simulink model "new16QAM"  (R2017b)
settings: Solver=VariableStepAuto  StartTime=0.0  StopTime=10.0  RelTol=1e-3
values from neighbouring files (symbols this model uses):
  Gain_lin = 10^(GdB/20)    [Microwave_Link.m]
  Var = 10^((N_dBm - 30)/10)    [Microwave_Link.m]
libraries: commblkcod2 x2, commdigbbndam3 x2, commchan3 x1, commsync2 x1, commsink2 x1, commrflib2 x1, commrandsrc3 x1
settings Model: Creator=m.s  LastModifiedBy=m.s

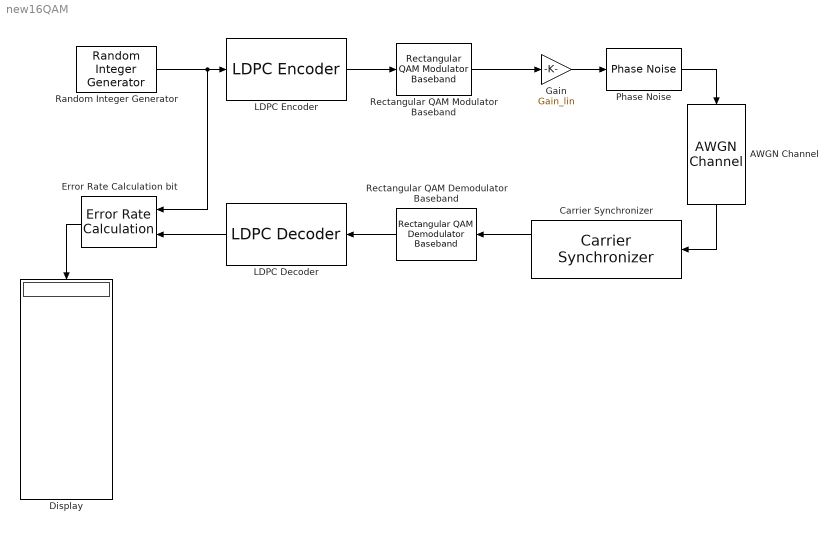
== system new16QAM ==
  AWGN Channel : commchan3/AWGN Channel  InputProcessing=Columns as channels (frame based)  seed=5  noiseMode=Variance from mask  EbNodB=6  EsNodB=10  SNRdB=55  bitsPerSym=1  Ps=1  Tsym=1  variance=Var
  Carrier Synchronizer : commsync2/Carrier Synchronizer  Modulation=QAM  ModulationPhaseOffset=Auto  CustomPhaseOffset=0  SamplesPerSymbol=1  DampingFactor=1  NormalizedLoopBandwidth=0.001  EstimatedPhaseErrorOutputPort=on  SimulateUsing=Code generation
      settings: SourceProductName=Communications System Toolbox
  Display : Display
  Error Rate Calculation bit : commsink2/Error Rate Calculation  N=0  st_delay=0  cp_mode=Entire frame  subframe=[]  PMode=Port  WsName=ErrorVec  RsMode2=off  stop=off  numErr=100  maxBits=1e6
  Gain : Gain  Gain=Gain_lin
  LDPC Decoder : commblkcod2/LDPC Decoder  ParityCheckMat=H  OutputFmt=Information part  DecisionType=Hard decision  OutputDataType=double  NumIter=50  DoParityCheck=on  OutputNumIter=off  OutputFinalChecks=off
      settings: SourceProductName=Communications System Toolbox  SourceProductBaseCode=CM
  LDPC Encoder : commblkcod2/LDPC Encoder  ParityCheckMat=H
      settings: SourceProductName=Communications System Toolbox  SourceProductBaseCode=CM
  Phase Noise : commrflib2/Phase Noise  PhNs=[-70 -90]  Fo=[1e3 1e6]  Fs=20e6  seed=2137
      settings: SourceProductName=Communications System Toolbox  SourceProductBaseCode=CM
  Random Integer Generator : commrandsrc3/Random Integer Generator  SetSize=2  SeedSource=Parameter  Seed=0  SampleTime=1  SamplesPerFrame=K  OutputDataType=double  SimulateUsing=Interpreted execution
  Rectangular QAM Demodulator Baseband : commdigbbndam3/Rectangular QAM Demodulator Baseband  M=16  OutType=Bit  DecType=Approximate log-likelihood ratio  VarSource=Dialog  Variance=Var  Dec=Gray  Mapping=[0:15]  PowType=Average Power  MinDist=2  AvgPow=1  PeakPow=1  Ph=0  outDtype1=Inherit via internal rule  outDtype2=Inherit via internal rule  derotateFactorWordLen=16  derotateFactorDataTypeStr=Inherit: Same word length as input  derotateFactorLastDataTypeStr=Inherit: Same word length as input  denormFactorWordLen=16  denormFactorDataTypeStr=Inherit: Same word length as input  denormFactorLastDataTypeStr=Inherit: Same word length as input  prodOutWordLen=32  prodOutOverflowMode=Wrap  prodOutRoundingMode=Floor  prodOutOvFlMode=off  prodOutOvFlModeLastStrValue=off  sumWordLen=32
  Rectangular QAM Modulator Baseband : commdigbbndam3/Rectangular QAM Modulator Baseband  M=16  InType=Bit  Enc=Gray  Mapping=[0:15]  PowType=Average Power  MinDist=2  AvgPow=1  PeakPow=1  Ph=0  outDtype=double  outWordLen=16  outUDDataType=sfix(16)  outFracLenMode=Best precision  outFracLen=15  outDataTypeStr=double  outLastDataTypeStr=double
  wires:
  Error Rate Calculation bit/1 -> Display/1
  Random Integer Generator/1 -> LDPC Encoder/1, Error Rate Calculation bit/1
  Gain/1 -> Phase Noise/1
  LDPC Decoder/1 -> Error Rate Calculation bit/2
  AWGN Channel/1 -> Carrier Synchronizer/1
  Phase Noise/1 -> AWGN Channel/1
  Rectangular QAM Modulator Baseband/1 -> Gain/1
  LDPC Encoder/1 -> Rectangular QAM Modulator Baseband/1
  Rectangular QAM Demodulator Baseband/1 -> LDPC Decoder/1
  Carrier Synchronizer/1 -> Rectangular QAM Demodulator Baseband/1
